simulink model "navigator_old"  (R2021a)
settings: Solver=VariableStepAuto  StartTime=0.0  StopTime=10.0  RelTol=1e-3
undefined symbols (not defined in the file or in its folder): NAV_ACC_RAD, RTL_CONE_ANG, RTL_LOITER_RAD, RTL_RETURN_ALT
settings Model: DataDictionary=px4_dict.sldd  Creator=DELL  LastModifiedBy=DELL

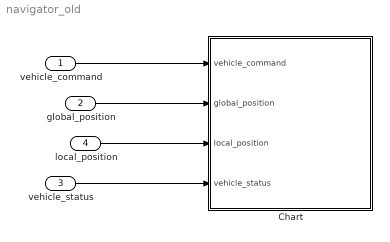
== system navigator_old ==
  vehicle_command : Inport  OutDataTypeStr=Bus: px4_vehicle_command
  global_position : Inport  Port=2  OutDataTypeStr=Bus: px4_vehicle_global_position
  vehicle_status : Inport  Port=3  OutDataTypeStr=Bus: px4_vehicle_status
  local_position : Inport  Port=4  OutDataTypeStr=Bus: px4_vehicle_local_position
  Chart : Stateflow chart  TreatAsAtomicUnit=on
  wires:
  vehicle_command/1 -> Chart/1(vehicle_command)
  global_position/1 -> Chart/2(global_position)
  local_position/1 -> Chart/3(local_position)
  vehicle_status/1 -> Chart/4(vehicle_status)

== stateflow chart navigator_old/Chart ==
  state LOITER
    state reposition
      en:
      % 当前位置作为上一个航路点
      position_sp_triplet.previous.lat = global_position.lat;
      position_sp_triplet.previous.lon = global_position.lon;
      position_sp_triplet.previous.alt = global_position.alt
      position_sp_triplet.previous.yaw = local_position.heading;
      % 当前航路点用rep中表示
      position_sp_triplet.current = reposition_triplte.current;
      position_sp_triplet.current.velocity_valid = false;
      % 下一个航路点无效
      position_sp_triplet.next.valid = false;
      % 设置reposition无效
      reposition_triplte.current.valid = false;
    state disarmed
    state loiternext
      en:
      mission_item = set_loiter_item(MIS_LTRMIN_ALT);
      % 上个航路
      position_sp_triplet.previous.valid = false;
      % 当前航点
      mission_item.nav_cmd = MAV_CMD.NAV_LOITER_UNLIMITED;
      mission_item.lat = position_sp_triplet.current.lat;
      mission_item.lon = position_sp_triplet.current.lon;
      mission_item.altitude = position_sp_triplet.current.alt;
      mission_item_to_position_setpoint
      % 下个航点
      position_sp_triplet.next.valid = false;
    state landed
      en,du:
      position_sp_triplet.current.type = PX4_POSITION_SETPOINT.SETPOINT_TYPE_IDLE;
    state loiterlocal
      en:
      mission_item = set_loiter_item(MIS_LTRMIN_ALT);
      % 上个航路
      position_sp_triplet.previous.valid = false;
      % 当前航点
      position_sp_triplet.current.velocity_valid = false;
      % 下个航点
      position_sp_triplet.next.valid = false;
    reposition -> reposition [order 2] : [reposition_triplte.current.valid]
    (default) -> (junction 105)
    (junction 105) -> reposition [order 1] : [reposition_triplte.current.valid]
    (junction 105) -> (junction 111) [order 2]
    reposition -> landed [order 1] : [land_detected]
    (junction 111) -> loiternext [order 1] : [position_sp_triplet.current.valid]
    (junction 111) -> (junction 109) [order 2]
    loiterlocal -> landed
    (junction 109) -> loiterlocal
  state vehicle_command
    state CMD_DO_GO_AROUND [parallel]
      settings: executionOrder=1
    state CMD_DO_REPOSITION [parallel]
      en:
      settings: executionOrder=2
    state CMD_NAV_TAKEOFF [parallel]
      settings: executionOrder=3
  state RTL
    en:
    get_rtl_alt_and_rad()
    en,du:
    % 计算到着陆点的距离
    destination_dist = get_distance_to_next_waypoint(destination.lat, destination.lon, global_position.lat, gloabl_position.lon)
    state RTL_STATE_CLIMB
      en,du:
      if vehicle_status.vehicle_type == PX4_VEHICLE_STATUS.VEHICLE_TYPE_ROTARY_WING
      % 如果多旋翼则直接爬升到给定高度
      mission_item.nav_cmd = uint16(MAV_CMD.NAV_WAYPOINT);
      else
      %如果是固定翼，则盘旋上升到给定高度
      mission_item.nav_cmd = uint16(MAV_CMD.NAV_LOITER_TO_ALT);
      end
      mission_item.lat = global_position.lat;
      mission_item.lon = global_position.lon;
      mission_item.altitude = 0;
      mission_item.altitude_is_relative = false;
      mission_item.yaw = local_position.heading;
      mission_item.acceptance_radius = single(get_acceptance_radius());
      mission_item.time_inside = 0;
      mission_item.autocontinue = true;
      mission_item.origin =uint8( PX4_MISSION_ORIGIN.ONBOARD);
      %mavlink_log_info(_navigator->get_mavlink_log_pub(), "RTL: climb to %d m (%d m above destination)\t",(int)ceilf(_rtl_alt), (int)ceilf(_rtl_alt - _destination.alt));
    state RTL_STATE_RETURN
      en,du:
      mission_item.nav_cmd = NAV_CMD.NAV_WAYPOINT;
      mission_item.lat = destination.lat;
      mission_item.lon = destination.lon;
      mission_item.altitude = 0;
      mission_item.altitude_is_relative = false;
      if destination_dist < RTL_MIN_DIST
      % 如果离着陆点很近，则采用着陆的航向
      mission_item.yaw = destination.yaw;
      else
      % 否则机头指向着陆点
      mission_item.yaw = get_bearing_to_next_waypoint(global_position.lat, global_position.lon, destination.lat, destination.lon)
      end
      mission_item.acceptance_radius = get_acceptance_radius();
      mission_item.time_inside = 0.0;
      mission_item.autocontinue = true;
      mission_item.origin = uint8(PX4_MISSION_ORIGIN.ONBOARD);
    state RTL_STATE_DESCEND
      en,du:
      mission_item.nav_cmd = uint16(MAV_CMD.NAV_LOITER_TO_ALT);
      mission_item.lat = destination.lat;
      mission_item.lon = destination.lon;
      mission_item.altitude = loiter_altitude;
      mission_item.altitude_is_relative = false;
      % Except for vtol which might be still off here and should point towards this location.
      d_current = get_distance_to_next_waypoint(global_position.lat, global_position.lon, mission_item.lat, mission_item.lon);
      if (vehicle_status.is_vtol && (d_current > get_acceptance_radius()))
      mission_item.yaw = get_bearing_to_next_waypoint(gpos.lat, gpos.lon, mission_item.lat, mission_item.lon);
      else
      mission_item.yaw = destination.yaw;
      end
      if (vehicle_status.is_vtol)
      mission_item.loiter_radius = rtl_loiter_rad;
      end
      mission_item.acceptance_radius = get_acceptance_radius();
      mission_item.time_inside = 0.0;
      mission_item.autocontinue = true;
      mission_item.origin = uint8(PX4_MISSION_ORIGIN.ONBOARD);
      % Disable previous setpoint to prevent drift.
      pos_sp_triplet.previous.valid = false;
    state RTL_STATE_LOITER
      en,du:
      autoland = RTL_LAND_DELAY > 0;
      % Don't change altitude.
      mission_item.lat = destination.lat;
      mission_item.lon = destination.lon;
      mission_item.altitude = loiter_altitude;
      mission_item.altitude_is_relative = false;
      mission_item.yaw = destination.yaw;
      mission_item.loiter_radius = get_loiter_radius();
      mission_item.acceptance_radius = get_acceptance_radius();
      mission_item.time_inside = max(RTL_LAND_DELAY, 0.0);
      mission_item.autocontinue = autoland;
      mission_item.origin = uint8(PX4_MISSION_ORIGIN.ONBOARD);
      set_can_loiter_at_sp(true);
      if (autoland)
      mission_item.nav_cmd = uint16(MAV_CMD.NAV_LOITER_TIME_LIMIT);
      %mavlink_log_info(_navigator->get_mavlink_log_pub(), "RTL: loiter %.1fs\t", (double)get_time_inside(_mission_item));
      %events::send<float>(events::ID("rtl_loiter"), events::Log::Info, "RTL: loiter {1:.1}s", get_time_inside(_mission_item));
      else
      mission_item.nav_cmd = uint16(MAV_CMD.NAV_LOITER_UNLIMITED);
      %mavlink_log_info(_navigator->get_mavlink_log_pub(), "RTL: completed, loitering\t");
      %events::send(events::ID("rtl_completed_loiter"), events::Log::Info, "RTL: completed, loitering");
      end
    state RTL_STATE_LAND
      en,du:
      % Land at destination.
      mission_item.nav_cmd = NAV_CMD_LAND;
      mission_item.lat = destination.lat;
      mission_item.lon = destination.lon;
      mission_item.yaw = destination.yaw;
      mission_item.altitude = destination.alt;
      mission_item.altitude_is_relative = false;
      mission_item.acceptance_radius = get_acceptance_radius();
      mission_item.time_inside = 0.0;
      mission_item.autocontinue = true;
      mission_item.origin = uint8(PX4_MISSION_ORIGIN.ONBOARD);
      mission_item.land_precision = RTL_PLD_MD;
      if (mission_item.land_precision == 1)
      %_navigator->get_precland()->set_mode(PrecLandMode::Opportunistic);
      %_navigator->get_precland()->on_activation();
      elseif (mission_item.land_precision == 2) {
      %_navigator->get_precland()->set_mode(PrecLandMode::Required);
      %_navigator->get_precland()->on_activation();
      end
      %mavlink_log_info(_navigator->get_mavlink_log_pub(), "RTL: land at destination\t");
      %events::send(events::ID("rtl_land_at_destination"), events::Log::Info, "RTL: land at destination");
    state RTL_MOVE_TO_LAND_HOVER_VTOL
      en,du:
      mission_item.nav_cmd = uint16(MAV_CMD.NAV_WAYPOINT);
      mission_item.lat = destination.lat;
      mission_item.lon = destination.lon;
      mission_item.altitude = loiter_altitude;
      mission_item.altitude_is_relative = false;
      mission_item.yaw = get_bearing_to_next_waypoint(global_position.lat, global_position.lon, mission_item.lat, mission_item.lon);
      mission_item.acceptance_radius = get_acceptance_radius();
      mission_item.origin = uint8(PX4_MISSION_ORIGIN.ONBOARD);
    state RTL_STATE_TRANSITION_TO_MC
      en,du:
      mission_item.nav_cmd = uint16(MAV_CMD.DO_VTOL_TRANSITION);
      mission_item.params(1) = single(VTOL_VEHICLE_STATUS.VEHICLE_VTOL_STATE_MC);
      mission_item.params(2) = 0.0;
      mission_item.yaw = local_position.heading;
      mission_item.autocontinue = true;
    state RTL_STATE_HEAD_TO_CENTER
    state RTL_STATE_LANDED
      en,du:
      mission_item.nav_cmd = uint16(0);
      mission_item.lat = home.lat;
      mission_item.lon = home.lon;
      mission_item.altitude_is_relative = false;
      mission_item.altitude = home.alt;
      mission_item.yaw = NaN;
      mission_item.loiter_radius = get_loiter_radius();
      mission_item.acceptance_radius = get_acceptance_radius();
      mission_item.time_inside = 0.0;
      mission_item.autocontinue = true;
      mission_item.origin = uint8(PX4_MISSION_ORIGIN.ONBOARD);
    (default) -> RTL_STATE_DESCEND [order 2] : [destination.type == PX4_RTL_DESTINATION_TYPE.MISSION_LANDING]
    (default) -> RTL_STATE_CLIMB [order 3] : [global_position.alt < destination.alt + RTL_RETURN_ALT ]
    (default) -> RTL_STATE_CLIMB [order 4]
    RTL_STATE_RETURN -> RTL_STATE_DESCEND : [is_mission_item_reached()]
    RTL_STATE_DESCEND -> RTL_STATE_LOITER
    RTL_STATE_CLIMB -> RTL_STATE_RETURN : [is_mission_item_reached()]
    RTL_STATE_LOITER -> RTL_STATE_HEAD_TO_CENTER
    RTL_STATE_HEAD_TO_CENTER -> RTL_STATE_TRANSITION_TO_MC
    RTL_STATE_TRANSITION_TO_MC -> RTL_MOVE_TO_LAND_HOVER_VTOL
    RTL_MOVE_TO_LAND_HOVER_VTOL -> RTL_STATE_LAND
    RTL_STATE_LAND -> RTL_STATE_LANDED
    (default) -> RTL_STATE_LANDED [order 1] : [landed]
  state GEOFENSE
  state TRAFFIC
  (default) -> vehicle_command
  data: item function_output; abs_altitude function_input; item function_output; item function_output; item function_output; at_current_location function_input; isreached function_output; item function_input; item function_input; pos_sp function_output; alt function_output single; item function_input; radius function_output single; throttle function_output single; radius function_output single; vehicle_command input; global_position input; local_position input; vehicle_status input; destination local Bus: px4_rtl_position size=1; landed local =false; RTL_RETURN_ALT parameter; RTL_CONE_ANG parameter; RTL_LOITER_RAD parameter; mission_item local Bus: px4_mission_item; NAV_ACC_RAD parameter
  function get_reposition_setpoint:
    | function get_reposition_setpoint
    | 
    | %% 判断reposition是否在禁飞区内
    | if GF_ACTION ~= PX4_GEOFENCE_RESULT.GF_ACTION_NONE &&  GF_ACTION ~= PX4_GEOFENCE_RESULT.GF_ACTION_WARN
    |     %mavlink_log_critical(&_mavlink_log_pub, "Reposition is outside geofence\t");
    |     %events::send(events::ID("navigator_reposition_outside_geofence"), {events::Log::Error, events::LogInternal::Info},
    |     %"Reposition is outside geofence");
    |     return;
    | end
    | 
    | 
    | %% 初始化上个航点
    | reposition_triplet.previous.valid = true;
    | reposition_triplet.previous.timestamp = hrt_absolute_time();
    | reposition_triplet.previous.lat = global_position.lat;
    | reposition_triplet.previous.lon = global_position.lon;
    | reposition_triplet.previous.alt = global_position.alt;
    | reposition_triplet.previous.yaw = local_position.heading;
    | 
    | %% 初始化当前航点
    | reposition_triplet.current.valid = true;
    | reposition_triplet.current.timestamp = hrt_absolute_time();
    | reposition_triplet.current.loiter_radius= get_loiter_radius();
    | reposition_triplet.current.loiter_direction = 1;
    | reposition_triplet.current.type = PX4_POSITION_SETPOINT.SETPOINT_TYPE_LOITER;
    | 
    | % 速度
    | if vehicle_command.param1 <= 0 || ~isfinite(vehicle_command.param1)
    |     reposition_triplet.current.cruising_speed = get_cruising_speed();
    | else
    |     reposition_triplet.current.cruising_speed = vehicle_command.param1;
    | end
    | % 油门
    | reposition_triplet.current.cruising_throttle = get_cruising_throttle();
    | % 接受半径
    | reposition_triplet.current.acceptance_radius = get_acceptance_radius();
    | % 偏航角
    | if isfinite(vehicle_command.param4)
    |     reposition_triplet.current.yaw = vehicle_command.param4;
    |     reposition_triplet.current.yaw_valid = true;
    | else
    |     reposition_triplet.current.yaw = NaN;
    |     reposition_triplet.current.yaw_valid = false;
    | end
    | % 经纬高
    | if isfinite(vehicle_command.param5) && isfinite(vehicle_command.param6)
    |     reposition_triplet.current.lat = vehicle_command.param5;
    |     reposition_triplet.current.lon = vehicle_command.param6;
    | elseif position_setpoint_triplet.current.valid
    |     reposition_triplet.current.lat = position_setpoint_triplet.current.lat;
    |     reposition_triplet.current.lon = position_setpoint_triplet.current.lon;
    | else
    |     % 如果是多旋翼会计算一个刹车距离，然后确定一个悬停位置
    |     
    |     % 固定翼直接使用当前位置进行盘旋
    |     reposition_triplet.current.lat = global_position.lat;
    |     reposition_triplet.current.lon = global_position.lon;
    |     reposition_triplet.current.alt = global_position.alt;
    | end
    | % 高度
    | if isfinite(vehicle_command.param7)
    |     reposition_triplet.current.alt = vehicle_command.param7;
    | else
    |     reposition_triplet.current.alt = global_position.alt;
    | end
    | 
    | %% 初始化下个航点
    | reposition_triplet.next.valid = false;
  function get_rtl_alt_and_rad:
    | function get_rtl_alt_and_rad
    | % 盘旋半径
    | % RTL_LOITER_RAD=1;
    | % RTL_CONE_ANG =1;
    | 
    | 
    | rtl_loiter_rad = RTL_LOITER_RAD;
    | % 
    | % % 返回高度
    | % if vehicle_status.vehicle_type == PX4_VEHICLE_STATUS.VEHICLE_TYPE_ROTARY_WING
    | %     rtl_alt = calculate_return_alt_from_cone_half_angle(RTL_CONE_ANG);
    | % else
    | %     rtl_alt = max(global_position.alt, destination.alt + RTL_RETURN_ALT);
    | % end
    | % 
    | % 
    | % function alt = calculate_return_alt_from_cone_half_angle(cone_half_angle_deg)
    | % 
    | % % horizontal distance to destination
    | % destination_dist = get_distance_to_next_waypoint(destination.lat, destination.lon, gloabl_position.lat, gloabl_position.lon);
    | % 
    | % % minium rtl altitude to use when outside of horizontal acceptance radius of target position.
    | % % We choose the minimum height to be two times the distance from the land position in order to
    | % % avoid the vehicle touching the ground while still moving horizontally.
    | % return_altitude_min_outside_acceptance_rad_amsl = destination.alt + 2.0 * get_acceptance_radius();
    | % 
    | % return_altitude_amsl = destination.alt + RTL_RETURN_ALT;
    | % 
    | % if (destination_dist <= get_acceptance_radius())
    | %     return_altitude_amsl = destination.alt + 2.0 * destination_dist;
    | %     
    | % else
    | %     if (cone_half_angle_deg > 0.0 && destination_dist <= RTL_MIN_DIST)
    | %         
    | %         % constrain cone half angle to meaningful values. All other cases are already handled above.
    | %         cone_half_angle_rad = deg2rad(min(max(cone_half_angle_deg, 1.0), 89.0));
    | %         
    | %         % minimum altitude we need in order to be within the user defined cone
    | %         cone_intersection_altitude_amsl = destination_dist / tan(cone_half_angle_rad) + destination.alt;
    | %         
    | %         return_altitude_amsl = min(cone_intersection_altitude_amsl, return_altitude_amsl);
    | %     end    
    | %     return_altitude_amsl = max(return_altitude_amsl, return_altitude_min_outside_acceptance_rad_amsl);
    | % end
    | % alt = max(return_altitude_amsl, gloabl_position.alt);
  function item = set_loiter_item:
    | function item = set_loiter_item
    |  
    | item.nav_cmd = MAV_CMD.NAV_LOITER_UNLIMITED;
  function item = set_takeoff_item(abs_altitude):
    | function item = set_takeoff_item(abs_altitude)
    |  
    | item.nav_cmd = MAV_CMD.NAV_TAKEOFF;
    | 
    | item.lat = global_position.lat;
    | item.lon = global_position.lon;
    | item.yaw = loacl_position.yaw;
    | item.altitude = abs_altitude;
    | item.altitude_is_relative = false;
    | 
    | item.loiter_radius = get_loiter_radius();
    | item.autocontinue = false;
    | item.origin = uint8(PX4_MISSION_ORIGIN.ONBOARD);
  function item = set_idle_item:
    | function item = set_idle_item
    | 
    | item.nav_cmd = uint16(MAV_CMD.IDLE);
    | item.lat = home.lat;
    | item.lon = home.lon;
    | item.altitude_is_relative = false;
    | item.altitude = home.alt;
    | item.yaw = NaN;
    | item.loiter_radius = get_loiter_radius();
    | item.acceptance_radius = get_acceptance_radius();
    | item.time_inside = 0.0;
    | item.autocontinue = true;
    | item.origin = uint8(PX4_MISSION_ORIGIN.ONBOARD);
  function item = set_land_item(at_current_location):
    | function item = set_land_item(at_current_location)
    | % if (_navigator.force_vtol())
    | %     
    | %     vehicle_command_s vcmd = {};
    | %     vcmd.command = NAV_CMD_DO_VTOL_TRANSITION;
    | %     vcmd.param1 = vtol_vehicle_status_s::VEHICLE_VTOL_STATE_MC;
    | %     vcmd.param2 = 0.0f;
    | %     _navigator.publish_vehicle_cmd(&vcmd);
    | % end
    | 
    | %/* set the land item */
    | item.nav_cmd = uint16(MAV_CMD.NAV_LAND);
    | 
    | %/* use current position */
    | if (at_current_location)
    |     item.lat = NaN; %descend at current position
    |     item.lon = NaN; %descend at current position
    |     item.yaw = local_position.heading;
    | else
    |     %/* use home position */
    |     item.lat = home.lat;
    |     item.lon = home.lon;
    |     item.yaw = home.yaw;
    | end
    | 
    | item.altitude = 0;
    | item.altitude_is_relative = false;
    | item.loiter_radius = get_loiter_radius();
    | item.acceptance_radius = get_acceptance_radius();
    | item.time_inside = 0.0;
    | item.autocontinue = true;
    | item.origin = uint8(PX4_MISSION_ORIGIN.ONBOARD);
  function isreached = is_item_reached(item):
    | function isreached = is_item_reached(item)
    | 
    | % 处理非导航指令
    | switch item.nav_cmd
    |     case MAV_CMD.DO_SET_SERVO
    |         isreached = true;
    |     case MAV_CMD.DO_CHANGE_SPEED
    |         isreached = true;
    |     case MAV_CMD.DO_SET_HOME
    |         isreached = true;
    | end
    | 
    | % 计算到目标点的距离
    | [dist, dist_xy, dist_z] = get_distance_to_point_global_wgs84(item.lat, item.lon, item.alt, ...
    |     global_position.lat, global_position.lon, global_position.alt);
    | 
    | 
    | %% yaw是否达到
    | if waypoint_position_reached && ~waypoint_yaw_reachead
    |     if vehicle_status.vehicle_type == PX4_VEHICLE_STATUS.VEHICLE_TYPE_ROTARY_WING && ...
    |             isfinite(item.yaw)
    |         % 多旋翼会判断yaw是否到达
    |         yaw_error = wrap_pi(item.yaw - local_position.heading);
    |      
    |         if abs(yaw_error) < MIS_YAW_ERR || ...
    |                 MIS_YAW_TMT > 0 && ~item.force_heading
    |             waypoint_yaw_reachead = true;
    |         end
    |         
    |         if ~waypoint_yaw_reachead && MIS_YAW_TMT > 0 && ...
    |                 hrt_elapsed_time(wp_positon_reached_time) > MIS_YAW_TMT
    |             % 设置mission失败
    |             %set_mission_failure_heading_timeout();
    |         end
    |     else
    |         % 固定翼不需要判断yaw是否到达
    |         waypoint_yaw_reachead = true;
    |     end
    | end
    | 
    | %% time是否达到
    | if waypoint_position_reached && waypoint_yaw_reached
    |     time_inside_reached = false;
    |     
    | end
    | 
    | 
    | end
  function pos_sp = mission_item_to_position_setpoint(item):
    | function pos_sp = mission_item_to_position_setpoint(item)
    | pos_sp.lat = item.lat;
    | pos_sp.lon = item.lon;
    | pos_sp.alt = get_absolute_altitude_for_item(item);
    | pos_sp.yaw = item.yaw;
    | pos_sp.yaw_valid = isfinite(item.yaw);
    | 
    | pos_sp.loiter_radius = saturation(item.loiter_radius, NAV_LOITER_RAD, NAV_LOITER_RAD);
    | 
    | pos_sp.loiter_direction = sign(item.loiter_radius);
    | 
    | 
    | switch item.nav_cmd
    |     case MAV_CMD.IDLE
    |         pos_sp.type = 0;
    |     case MAV_CMD.NAV_TAKEOFF
    | end
  function alt = get_absolute_altitude_for_item(item):
    | function alt = get_absolute_altitude_for_item(item)
    | 
    | if item.altitude_is_relative
    |     alt = home.alt + item.altitude;
    | else
    |     alt = item.altitude;
    | end
  function radius = get_acceptance_radius:
    | function radius = get_acceptance_radius
    | radius = NAV_ACC_RAD;
    | 
    | 
    | % 	const position_controller_status_s &pos_ctrl_status = _position_controller_status_sub.get();
    | %
    | % 	// for fixed-wing and rover, return the max of NAV_ACC_RAD and the controller acceptance radius (e.g. L1 distance)
    | % 	if (_vstatus.vehicle_type != vehicle_status_s::VEHICLE_TYPE_ROTARY_WING
    | % 	    && PX4_ISFINITE(pos_ctrl_status.acceptance_radius) && pos_ctrl_status.timestamp != 0) {
    | %
    | % 		acceptance_radius = math::max(acceptance_radius, pos_ctrl_status.acceptance_radius);
    | % 	}
  function throttle = get_cruising_throttle:
    | function throttle = get_cruising_throttle
    | 
    | throttle = single(0.0);
    | 
    | % pos_ctrl_status = position_controller_status_sub.get();
    | 
    | % for fixed-wing and rover, return the max of NAV_ACC_RAD and the controller acceptance radius (e.g. L1 distance)
    | % if (vehicle_status.vehicle_type ~= PX4_VEHICLE_STATUS.VEHICLE_TYPE_ROTARY_WING && ...
    | %         isfinite(pos_ctrl_status.acceptance_radius) && pos_ctrl_status.timestamp ~= 0)
    | %     
    | %     radius = max(radius, pos_ctrl_status.acceptance_radius);
    | % end
  function radius = get_altitude_acceptance_radius:
    | function radius = get_altitude_acceptance_radius
    | switch vehicle_status.vehicle_type
    |     case PX4_VEHICLE_STATUS.VEHICLE_TYPE_FIXED_WING
    |         if (position_sp_triplet.next.type == PX4_POSITION_SETPOINT.SETPOINT_TYPE_LAND && position_sp_triplet.next.valid)
    |             %Use separate (tighter) altitude acceptance for clean altitude starting point before landing
    |             radius = NAV_FW_ALTL_RAD;
    |         else
    |             radius = NAV_FW_ALT_RAD;
    |         end
    |     case PX4_VEHICLE_STATUS.VEHICLE_TYPE_ROTARY_WING
    |         radius = NAV_FW_ALT_RAD;
    |         %         const position_controller_status_s &pos_ctrl_status = _position_controller_status_sub.get();
    |         %
    |         % 		if ((pos_ctrl_status.timestamp > _pos_sp_triplet.timestamp)
    |         % 		    && pos_ctrl_status.altitude_acceptance > alt_acceptance_radius) {
    |         % 			alt_acceptance_radius = pos_ctrl_status.altitude_acceptance;
    |         % 		}
    |     case PX4_VEHICLE_STATUS.VEHICLE_TYPE_ROVER
    |         radius = inf;
    |     otherwise
    |         radius = NaN;
    | end
